simulink model "tailsitter_simulation_main"  (R2021a)
settings: Solver=VariableStepAuto  StartTime=0.0  StopTime=tf  RelTol=1e-3
values from neighbouring files (symbols this model uses):
  b = 0.6    [simulink_setup.m]
  c_bar = 0.142    [simulink_setup.m]
  CD_f = 0.000762    [simulink_setup.m]
  CL_0 = 0    [simulink_setup.m]
  CL_f = 0.036    [simulink_setup.m]
  Cl_f = 0.0057    [simulink_setup.m]
  Cm_0 = 0    [simulink_setup.m]
  Cm_f = -0.0102    [simulink_setup.m]
  CP = 0.01    [simulink_setup.m]
  CT = 0.05    [simulink_setup.m]
  D = 0.12    [simulink_setup.m]
  g = 9.81    [simulink_setup.m]
  J = [Jxx 0 -Jxz; 0 Jyy 0; -Jxz 0 Jzz]    [simulink_setup.m]
  Kp = 10    [simulink_setup.m]
  Kq = 10    [simulink_setup.m]
  Kr = 10    [simulink_setup.m]
  Kt = -5    [simulink_setup.m]
  m = 0.3    [simulink_setup.m]
  M_flap = [-1 1; -1 -1]    [simulink_setup.m]
  M_motor = [1 1; 1 -1]    [simulink_setup.m]
  motor_eq = xeq(end)    [simulink_setup.m]
  prop_arm = 0.15    [simulink_setup.m]
  rho = 1.225    [simulink_setup.m]
  S_w = 0.0828    [simulink_setup.m]
libraries: sharedtransform x4, vrlib x3, aerolibutil x2, simulink_extras x1
settings Model: Creator=Owner  LastModifiedBy=Owner

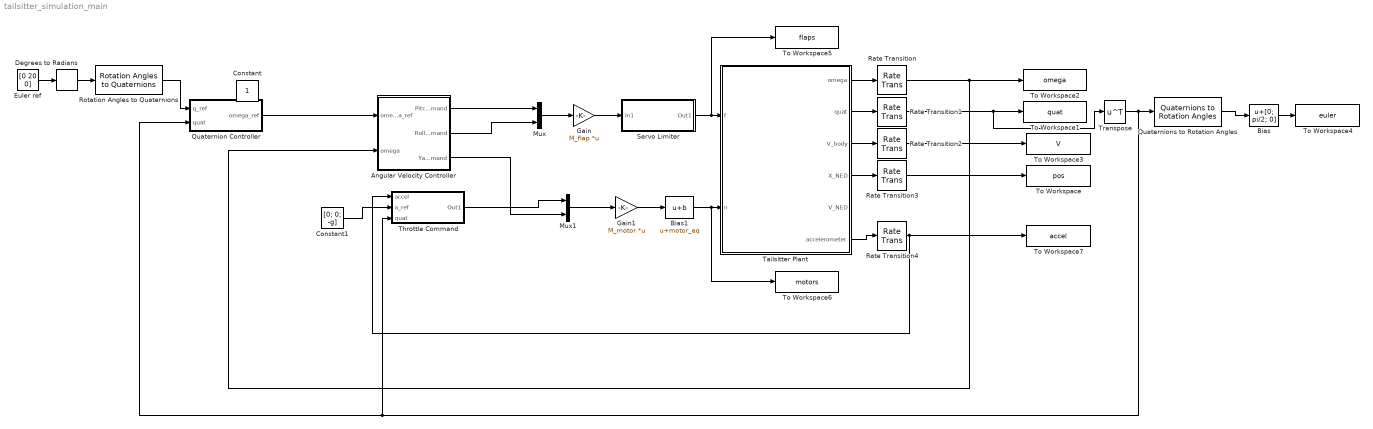
== system tailsitter_simulation_main ==
  Angular Velocity Controller : Subsystem
  Bias : Bias  Bias=[0; pi/2; 0]
  Bias1 : Bias  Bias=motor_eq
  Constant1 : Constant  Value=[0; 0; -g]
  Degrees to Radians : simulink_extras/Transformations/Degrees to Radians
  Euler ref : Constant  Value=[0 20 0]
  Gain : Gain  Gain=M_flap  Multiplication=Matrix(K*u)
  Gain1 : Gain  Gain=M_motor  Multiplication=Matrix(K*u)
  Mux : Mux  Inputs=2
  Mux1 : Mux  Inputs=2
  Quaternion Controller : Subsystem
  Quaternions to Rotation Angles : sharedtransform/Quaternions to Rotation Angles  rotationOrder=ZYX  aMode=aMode
      settings: SourceProductBaseCode=AE,PW,DR,MT,UV,VE
  Rate Transition{,1..3} (4 alike) : RateTransition  OutPortSampleTime=dt
  Rate Transition4 : RateTransition  OutPortSampleTime=0.005
  Rotation Angles to Quaternions : sharedtransform/Rotation Angles to Quaternions  rotationOrder=ZYX  aMode=aMode
      settings: SourceProductBaseCode=AE,PW,DR,MT,UV,VE
  Servo Limiter : Subsystem
  Tailsitter Plant : Subsystem
  Throttle Command : Subsystem
  To Workspace : ToWorkspace  VariableName=pos  SampleTime=-1
  To Workspace1 : ToWorkspace  VariableName=quat  SampleTime=-1
  To Workspace2 : ToWorkspace  VariableName=omega  SampleTime=-1
  To Workspace3 : ToWorkspace  VariableName=V  SampleTime=-1
  To Workspace4 : ToWorkspace  VariableName=euler  SampleTime=-1
  To Workspace5 : ToWorkspace  VariableName=flaps  SampleTime=-1
  To Workspace6 : ToWorkspace  VariableName=motors  SampleTime=-1
  To Workspace7 : ToWorkspace  VariableName=accel  SampleTime=-1
  Transpose : Math  Operator=transpose  SaturateOnIntegerOverflow=on
  Constant : Constant  IOType=siggen
  wires:
  Tailsitter Plant/4(X_NED) -> Rate Transition3/1
  Tailsitter Plant/1(omega) -> Rate Transition/1
  Tailsitter Plant/2(quat) -> Rate Transition1/1
  Tailsitter Plant/3(V_body) -> Rate Transition2/1
  Transpose/1 -> Throttle Command/3(quat), Quaternion Controller/2(quat), Quaternions to Rotation Angles/1
  Quaternions to Rotation Angles/1 -> Bias/1
  Bias/1 -> To Workspace4/1
  Gain1/1 -> Bias1/1
  Gain/1 -> Servo Limiter/1(In1)
  Quaternion Controller/1(omega_ref) -> Angular Velocity Controller/1(omega_ref)
  Angular Velocity Controller/1(Pitch Command) -> Mux/1
  Angular Velocity Controller/2(Roll Command) -> Mux/2
  Mux/1 -> Gain/1
  Angular Velocity Controller/3(Yaw Command) -> Mux1/2
  Mux1/1 -> Gain1/1
  Throttle Command/1(Out1) -> Mux1/1
  Tailsitter Plant/6(accelerometer) -> Rate Transition4/1
  Constant1/1 -> Throttle Command/2(a_ref)
  Rotation Angles to Quaternions/1 -> Quaternion Controller/1(q_ref)
  Degrees to Radians/1 -> Rotation Angles to Quaternions/1
  Euler ref/1 -> Degrees to Radians/1
  Rate Transition/1 -> Angular Velocity Controller/2(omega), To Workspace2/1
  Rate Transition1/1 -> Transpose/1, To Workspace1/1
  Rate Transition2/1 -> To Workspace3/1
  Rate Transition3/1 -> To Workspace/1
  Rate Transition4/1 -> Throttle Command/1(accel), To Workspace7/1
  Bias1/1 -> To Workspace6/1, Tailsitter Plant/2(n)
  Servo Limiter/1(Out1) -> To Workspace5/1, Tailsitter Plant/1(f)

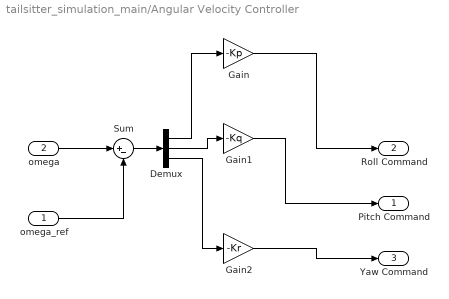
== system tailsitter_simulation_main/Angular Velocity Controller ==
  omega_ref : Inport
  omega : Inport  Port=2
  Demux : Demux  Outputs=3
  Gain : Gain  Gain=-Kp
  Gain1 : Gain  Gain=-Kq
  Gain2 : Gain  Gain=-Kr
  Sum : Sum  Inputs=|+-
  Pitch Command : Outport
  Roll Command : Outport  Port=2
  Yaw Command : Outport  Port=3
  wires:
  omega_ref/1 -> Sum/2
  omega/1 -> Sum/1
  Sum/1 -> Demux/1
  Demux/1 -> Gain/1
  Demux/2 -> Gain1/1
  Demux/3 -> Gain2/1
  Gain/1 -> Roll Command/1
  Gain2/1 -> Yaw Command/1
  Gain1/1 -> Pitch Command/1

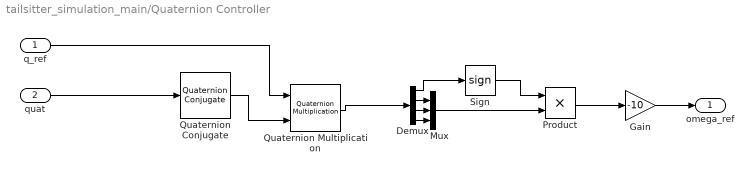
== system tailsitter_simulation_main/Quaternion Controller ==
  q_ref : Inport
  quat : Inport  Port=2
  Demux : Demux
  Gain : Gain  Gain=-10
  Mux : Mux  Inputs=3
  Product : Product
  Quaternion Conjugate : aerolibutil/Quaternion Conjugate
      settings: SourceProductBaseCode=AE
  Quaternion Multiplication : aerolibutil/Quaternion Multiplication
  Sign : Signum
  omega_ref : Outport
  wires:
  Quaternion Conjugate/1 -> Quaternion Multiplication/2
  q_ref/1 -> Quaternion Multiplication/1
  Quaternion Multiplication/1 -> Demux/1
  quat/1 -> Quaternion Conjugate/1
  Product/1 -> Gain/1
  Demux/1 -> Sign/1
  Sign/1 -> Product/1
  Gain/1 -> omega_ref/1
  Demux/2 -> Mux/1
  Demux/3 -> Mux/2
  Demux/4 -> Mux/3
  Mux/1 -> Product/2

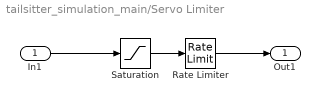
== system tailsitter_simulation_main/Servo Limiter ==
  In1 : Inport
  Rate Limiter : RateLimiter  RisingSlewLimit=400  FallingSlewLimit=-400  SampleTimeMode=inherited
  Saturation : Saturate  UpperLimit=20  LowerLimit=20
  Out1 : Outport
  wires:
  In1/1 -> Saturation/1
  Saturation/1 -> Rate Limiter/1
  Rate Limiter/1 -> Out1/1

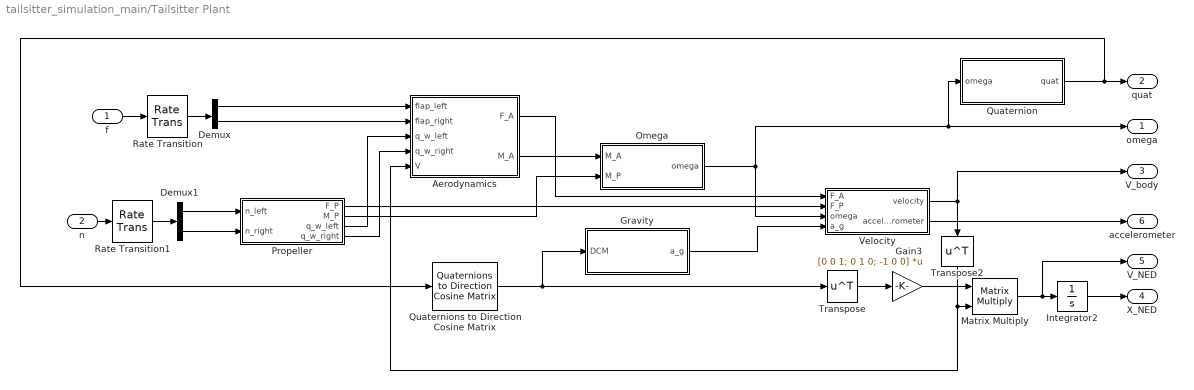
== system tailsitter_simulation_main/Tailsitter Plant ==
  f : Inport
  n : Inport  Port=2
  Aerodynamics : Subsystem
  Demux : Demux  Outputs=2
  Demux1 : Demux  Outputs=2
  Gain3 : Gain  Gain=[0 0 1; 0 1 0; -1 0 0]  Multiplication=Matrix(K*u)
  Gravity : Subsystem
  Integrator2 : Integrator
  Matrix Multiply : Product  Multiplication=Matrix(*)
  Omega : Subsystem
  Propeller : Subsystem
  Quaternion : Subsystem
  Quaternions to Direction Cosine Matrix : sharedtransform/Quaternions to  Direction Cosine Matrix  aMode=aMode
      settings: SourceProductBaseCode=AE,PW,DR,MT,UV,VE
  Rate Transition : RateTransition
  Rate Transition1 : RateTransition
  Transpose : Math  Operator=transpose  SaturateOnIntegerOverflow=on
  Transpose2 : Math  Operator=transpose  SaturateOnIntegerOverflow=on
  Velocity : Subsystem
  omega : Outport
  quat : Outport  Port=2
  V_body : Outport  Port=3
  X_NED : Outport  Port=4
  V_NED : Outport  Port=5
  accelerometer : Outport  Port=6
  wires:
  f/1 -> Rate Transition/1
  Aerodynamics/1(F_A) -> Velocity/1(F_A)
  Demux/1 -> Aerodynamics/1(flap_left)
  Demux/2 -> Aerodynamics/2(flap_right)
  Propeller/3(q_w_left) -> Aerodynamics/3(q_w_left)
  Demux1/1 -> Propeller/1(n_left)
  Demux1/2 -> Propeller/2(n_right)
  Propeller/4(q_w_right) -> Aerodynamics/4(q_w_right)
  Propeller/2(M_P) -> Omega/2(M_P)
  Quaternions to Direction Cosine Matrix/1 -> Transpose/1, Gravity/1(DCM)
  Gain3/1 -> Matrix Multiply/1
  Transpose/1 -> Gain3/1
  Matrix Multiply/1 -> V_NED/1, Integrator2/1
  Integrator2/1 -> X_NED/1
  n/1 -> Rate Transition1/1
  Omega/1(omega) -> Quaternion/1(omega), omega/1, Velocity/3(omega)
  Aerodynamics/2(M_A) -> Omega/1(M_A)
  Velocity/1(velocity) -> V_body/1, Transpose2/1
  Velocity/2(accelerometer) -> accelerometer/1
  Gravity/1(a_g) -> Velocity/4(a_g)
  Propeller/1(F_P) -> Velocity/2(F_P)
  Quaternion/1(quat) -> Quaternions to Direction Cosine Matrix/1, quat/1
  Transpose2/1 -> Aerodynamics/5(V), Matrix Multiply/2
  Rate Transition/1 -> Demux/1
  Rate Transition1/1 -> Demux1/1

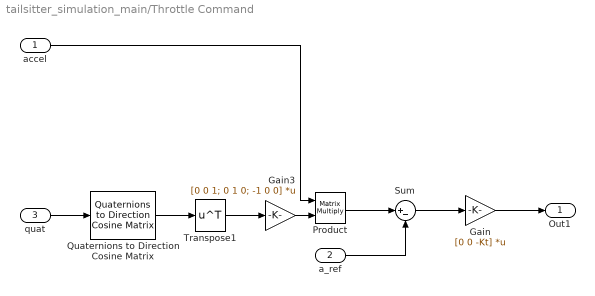
== system tailsitter_simulation_main/Throttle Command ==
  accel : Inport
  a_ref : Inport  Port=2
  quat : Inport  Port=3
  Gain : Gain  Gain=[0 0 -Kt]  Multiplication=Matrix(K*u) (u vector)
  Gain3 : Gain  Gain=[0 0 1; 0 1 0; -1 0 0]  Multiplication=Matrix(K*u)
  Product : Product  Multiplication=Matrix(*)
  Quaternions to Direction Cosine Matrix : sharedtransform/Quaternions to  Direction Cosine Matrix  aMode=aMode
      settings: SourceProductBaseCode=AE,PW,DR,MT,UV,VE
  Sum : Sum  Inputs=|+-
  Transpose1 : Math  Operator=transpose  SaturateOnIntegerOverflow=on
  Out1 : Outport
  wires:
  quat/1 -> Quaternions to Direction Cosine Matrix/1
  Quaternions to Direction Cosine Matrix/1 -> Transpose1/1
  Transpose1/1 -> Gain3/1
  Gain3/1 -> Product/2
  accel/1 -> Product/1
  a_ref/1 -> Sum/2
  Product/1 -> Sum/1
  Sum/1 -> Gain/1
  Gain/1 -> Out1/1

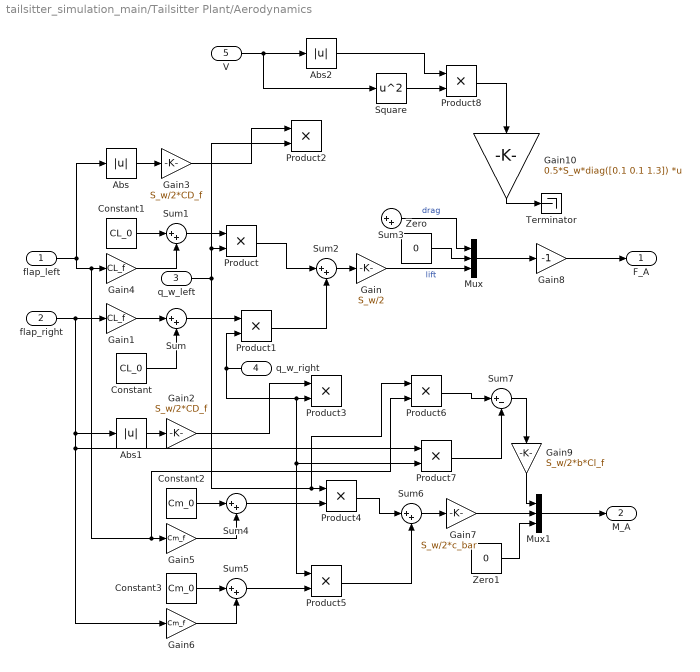
== system tailsitter_simulation_main/Tailsitter Plant/Aerodynamics ==
  flap_left : Inport
  flap_right : Inport  Port=2
  q_w_left : Inport  Port=3
  q_w_right : Inport  Port=4
  V : Inport  Port=5
  Abs : Abs
  Abs1 : Abs
  Abs2 : Abs
  Constant : Constant  Value=CL_0
  Constant1 : Constant  Value=CL_0
  Constant2 : Constant  Value=Cm_0
  Constant3 : Constant  Value=Cm_0
  Gain : Gain  Gain=S_w/2
  Gain1 : Gain  Gain=CL_f
  Gain10 : Gain  Gain=0.5*S_w*diag([0.1 0.1 1.3])  Multiplication=Matrix(K*u) (u vector)
  Gain2 : Gain  Gain=S_w/2*CD_f
  Gain3 : Gain  Gain=S_w/2*CD_f
  Gain4 : Gain  Gain=CL_f
  Gain5 : Gain  Gain=Cm_f
  Gain6 : Gain  Gain=Cm_f
  Gain7 : Gain  Gain=S_w/2*c_bar
  Gain8 : Gain  Gain=-1
  Gain9 : Gain  Gain=S_w/2*b*Cl_f
  Mux : Mux  Inputs=3
  Mux1 : Mux  Inputs=3
  Product{,1..8} (9 alike) : Product
  Square : Math  Operator=square  SaturateOnIntegerOverflow=on
  Sum{,1..6} (7 alike) : Sum  Inputs=|++
  Sum7 : Sum  Inputs=|+-
  Terminator : Terminator
  Zero : Constant  Value=0  OutDataTypeStr=Inherit: Inherit via back propagation
  Zero1 : Constant  Value=0  OutDataTypeStr=Inherit: Inherit via back propagation
  F_A : Outport
  M_A : Outport  Port=2
  wires:
  Gain1/1 -> Sum/1
  Constant/1 -> Sum/2
  Constant1/1 -> Sum1/1
  Gain4/1 -> Sum1/2
  Sum2/1 -> Gain/1
  Sum1/1 -> Product/1
  q_w_left/1 -> Product6/1, Product4/1, Product2/2, Product/2
  Sum/1 -> Product1/1
  q_w_right/1 -> Product1/2, Product7/2, Product5/1, Product3/2
  Product1/1 -> Sum2/2
  Product/1 -> Sum2/1
  Gain/1 -> Mux/3  "lift"
  Zero/1 -> Mux/2
  Abs1/1 -> Gain2/1
  Abs/1 -> Gain3/1
  Gain3/1 -> Product2/1
  Gain2/1 -> Product3/1
  Sum3/1 -> Mux/1  "drag"
  Constant2/1 -> Sum4/1
  flap_left/1 -> Abs/1, Product6/2, Gain5/1, Gain4/1
  Gain5/1 -> Sum4/2
  Gain6/1 -> Sum5/2
  Constant3/1 -> Sum5/1
  flap_right/1 -> Gain6/1, Product7/1, Abs1/1, Gain1/1
  Sum5/1 -> Product5/2
  Sum4/1 -> Product4/2
  Product4/1 -> Sum6/1
  Product5/1 -> Sum6/2
  Sum6/1 -> Gain7/1
  Mux1/1 -> M_A/1
  Gain7/1 -> Mux1/2
  Zero1/1 -> Mux1/3
  Gain8/1 -> F_A/1
  Gain9/1 -> Mux1/1
  Sum7/1 -> Gain9/1
  Product6/1 -> Sum7/1
  Product7/1 -> Sum7/2
  V/1 -> Square/1, Abs2/1
  Square/1 -> Product8/2
  Abs2/1 -> Product8/1
  Product8/1 -> Gain10/1
  Mux/1 -> Gain8/1
  Gain10/1 -> Terminator/1

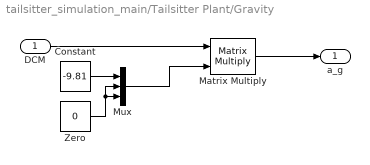
== system tailsitter_simulation_main/Tailsitter Plant/Gravity ==
  DCM : Inport
  Constant : Constant  Value=-9.81
  Matrix Multiply : Product  Multiplication=Matrix(*)
  Mux : Mux  Inputs=3
  Zero : Constant  Value=0  OutDataTypeStr=Inherit: Inherit via back propagation
  a_g : Outport
  wires:
  Mux/1 -> Matrix Multiply/2
  Constant/1 -> Mux/1
  Zero/1 -> Mux/3, Mux/2
  Matrix Multiply/1 -> a_g/1
  DCM/1 -> Matrix Multiply/1

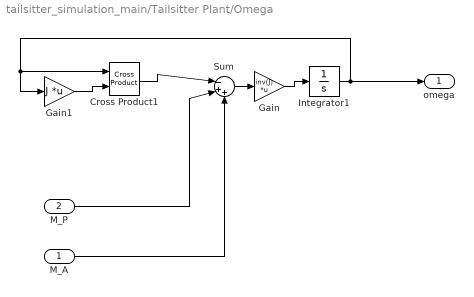
== system tailsitter_simulation_main/Tailsitter Plant/Omega ==
  M_A : Inport
  M_P : Inport  Port=2
  Cross Product1 : vrlib/Utilities/Cross Product
  Gain : Gain  Gain=inv(J)  Multiplication=Matrix(K*u) (u vector)
  Gain1 : Gain  Gain=J  Multiplication=Matrix(K*u) (u vector)
  Integrator1 : Integrator
  Sum : Sum  Inputs=|-++
  omega : Outport
  wires:
  Sum/1 -> Gain/1
  Cross Product1/1 -> Sum/1
  M_P/1 -> Sum/2
  Integrator1/1 -> omega/1, Cross Product1/1, Gain1/1
  Gain1/1 -> Cross Product1/2
  Gain/1 -> Integrator1/1
  M_A/1 -> Sum/3

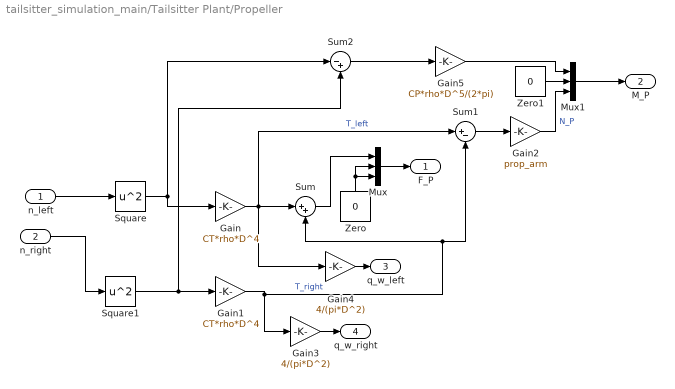
== system tailsitter_simulation_main/Tailsitter Plant/Propeller ==
  n_left : Inport
  n_right : Inport  Port=2
  Gain : Gain  Gain=CT*rho*D^4
  Gain1 : Gain  Gain=CT*rho*D^4
  Gain2 : Gain  Gain=prop_arm
  Gain3 : Gain  Gain=4/(pi*D^2)
  Gain4 : Gain  Gain=4/(pi*D^2)
  Gain5 : Gain  Gain=CP*rho*D^5/(2*pi)
  Mux : Mux  Inputs=3
  Mux1 : Mux  Inputs=3
  Square : Math  Operator=square  SaturateOnIntegerOverflow=on
  Square1 : Math  Operator=square  SaturateOnIntegerOverflow=on
  Sum : Sum  Inputs=|++
  Sum1 : Sum  Inputs=|+-
  Sum2 : Sum  Inputs=|-+
  Zero : Constant  Value=0  OutDataTypeStr=Inherit: Inherit via back propagation
  Zero1 : Constant  Value=0  OutDataTypeStr=Inherit: Inherit via back propagation
  F_P : Outport
  M_P : Outport  Port=2
  q_w_left : Outport  Port=3
  q_w_right : Outport  Port=4
  wires:
  Gain/1 -> Sum1/1, Gain4/1, Sum/1  "T_left"
  Gain1/1 -> Gain3/1, Sum/2, Sum1/2  "T_right"
  n_right/1 -> Square1/1
  Gain3/1 -> q_w_right/1
  n_left/1 -> Square/1
  Gain4/1 -> q_w_left/1
  Mux/1 -> F_P/1
  Sum/1 -> Mux/1
  Zero/1 -> Mux/3, Mux/2
  Mux1/1 -> M_P/1
  Zero1/1 -> Mux1/2
  Gain2/1 -> Mux1/3  "N_P"
  Sum1/1 -> Gain2/1
  Gain5/1 -> Mux1/1
  Square/1 -> Gain/1, Sum2/1
  Square1/1 -> Sum2/2, Gain1/1
  Sum2/1 -> Gain5/1

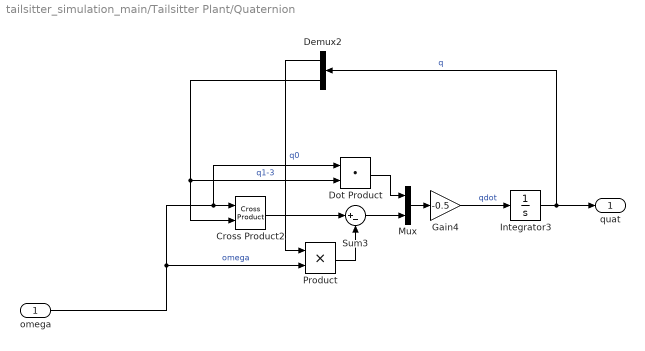
== system tailsitter_simulation_main/Tailsitter Plant/Quaternion ==
  omega : Inport
  Cross Product2 : vrlib/Utilities/Cross Product
  Demux2 : Demux  Outputs=2
  Dot Product : DotProduct  InputSameDT=on  OutDataTypeStr=Inherit: Inherit via internal rule
  Gain4 : Gain  Gain=-0.5
  Integrator3 : Integrator  InitialCondition=[1; 0; 0; 0]
  Mux : Mux  Inputs=2
  Product : Product
  Sum3 : Sum  Inputs=|+-
  quat : Outport
  wires:
  Integrator3/1 -> quat/1, Demux2/1  "q"
  Demux2/1 -> Product/1  "q0"
  omega/1 -> Product/2, Cross Product2/1, Dot Product/1  "omega"
  Dot Product/1 -> Mux/1
  Gain4/1 -> Integrator3/1  "qdot"
  Sum3/1 -> Mux/2
  Demux2/2 -> Cross Product2/2, Dot Product/2  "q1-3"
  Mux/1 -> Gain4/1
  Cross Product2/1 -> Sum3/1
  Product/1 -> Sum3/2

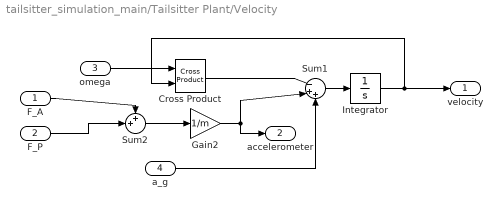
== system tailsitter_simulation_main/Tailsitter Plant/Velocity ==
  F_A : Inport
  F_P : Inport  Port=2
  omega : Inport  Port=3
  a_g : Inport  Port=4
  Cross Product : vrlib/Utilities/Cross Product
  Gain2 : Gain  Gain=1/m
  Integrator : Integrator
  Sum1 : Sum  Inputs=|-++
  Sum2 : Sum  Inputs=++|
  velocity : Outport
  accelerometer : Outport  Port=2
  wires:
  Sum2/1 -> Gain2/1
  F_A/1 -> Sum2/1
  Gain2/1 -> accelerometer/1, Sum1/2
  a_g/1 -> Sum1/3
  Sum1/1 -> Integrator/1
  F_P/1 -> Sum2/2
  omega/1 -> Cross Product/1
  Cross Product/1 -> Sum1/1
  Integrator/1 -> Cross Product/2, velocity/1
